simulink model "TRN_V3_2_CodeGen"  (R2022a)
settings: Solver=FixedStepAuto  StartTime=0.0  StopTime=300  FixedStep=0.04  RelTol=1e-3
PreLoadFcn:
  | load('BusStructureTRNsensor.mat');
  | addpath('C:/MAP');
InitFcn:
  | %load TRNDataBusPILS.mat
  | %addpath(genpath(cd))
  | 
  | %load('TPF_WHOLESIM_INPUT_SCENARIOS_AGCAS_N35_10E127_70.mat');
  | 
  | % Add DataBus Path
  | addpath(',,/');
  | addpath('../MAP/');
  | addpath('../MAP/MAP_DB');
  | addpath('../MAP/DVOF');
  | addpath(genpath(cd));
  | load('BusStructureTRN.mat');
undefined symbols (not defined in the file or in its folder): Altitude_INS, Latitude_INS, Longitude_INS, TRN, TRNlib
libraries: simulink_extras x23, aerolibconvert2 x6, sharedtransform x4, dspstat3 x2
(part 3 of 3)

== stateflow chart TRN_V3_2_CodeGen/TRN/ModeManagementCSU_v6 ==
  state Operation_In_Flight
    state Terrain_Referenced_Navigation [parallel]
      settings: executionOrder=1
      state TrackingCSU
        state ContinuousUpdate [parallel]
          en,du:
          [INS_Lat,INS_Lon,INS_Alt,Out_TRNDatapump.TimeTag_Prev] = TrackingCSUTimeTag(In_TRNDatapump,In_TRNInput);
          [Fmatrix,Gmatrix,M,N] = FmatGmatUpdate(INS_Lat,INS_Alt,In_TRNInput);
          [Hmat_TRN,zmat_TRN,Rmat_TRN,Hmat_GPS,zmat_GPS,Rmat_GPS, GPSflag] = ...
          TrackingCSUMeasurement(In_TRNInput,In_TRNDatapump,INS_Lat,INS_Lon,INS_Alt,M,N);
          [Out_TRNDatapump.xu, Out_Pmatrix, Out_TRNDatapump.residual, latINSErrTRN, lonINSErrTRN, altINSErrTRN,...
          Out_TRNOutput.TRNHorUncertainty, Out_TRNOutput.TRNVerticalUncertainty] ...
          = TrackingCSUEKFUpdate(In_TRNInput, zmat_TRN, zmat_GPS, Fmatrix, Hmat_TRN, Hmat_GPS, Gmatrix, In_Pmatrix, ...
          Qmatrix, Rmat_TRN, Rmat_GPS, GPSflag, Out_TRNDatapump);
          [continuousValid, Out_TRNOutput.NavigationMode]...
          = CheckValidity( Out_TRNOutput.TRNHorUncertainty, In_TRNInput.INSDataNotValid, In_TRNInput.INS_Alignment_State, ...
          In_TRNInput.GPSDataNotValid);
          [Out_TRNOutput.TRN_Ver_FlightPath_Angle] = Ver_FlightPath_Angle(In_TRNInput);
          settings: executionOrder=1
        state ContinuousValid [parallel]
          en, du:
          [Out_TRNOutput.TRNEstOfINSLatitudeErr, Out_TRNOutput.TRNEstOfINSLongitudeErr, Out_TRNOutput.TRNEstOfINSAltitudeErr, ...
          Out_TRNOutput.AircraftPositionCorrectionValid] = ValidityCheck(continuousValid, latINSErrTRN, lonINSErrTRN, altINSErrTRN);
          settings: executionOrder=2
      state AcquisitionCSU
        state Batch_On
          state StoreProfile [parallel]
            en, du: [Out_TRNDatapump.profileCnt] = StoreProfile(In_TRNInput, In_TRNDatapump);
            SetProfile(In_TRNDatapump, In_TRNInput);
            CollectProfile(Out_TRNDatapump);
            [posUpdate, Out_TRNDatapump.MAD, Out_TRNDatapump.residual] = CorrelationAnalysis(Out_TRNDatapump);
            settings: executionOrder=1
          state BatchUpdate_Valid [parallel]
            en, du:
            [Out_TRNOutput.TRNEstOfINSLatitudeErr, Out_TRNOutput.TRNEstOfINSLongitudeErr, Out_TRNOutput.TRNEstOfINSAltitudeErr, ...
            Out_TRNDatapump.profileCnt, Out_TRNOutput.NavigationMode, Out_TRNOutput.AircraftPositionCorrectionValid ] = ...
            CorrelationValid(Out_TRNDatapump, In_TRNInput, posUpdate);
            [Out_TRNOutput.TRN_Ver_FlightPath_Angle] = Ver_FlightPath_Angle(In_TRNInput);
            Out_Pmatrix = InitPmatrix();
            settings: executionOrder=2
        state Batch_Idle
          entry: Out_TRNOutput.TRNEstOfINSLatitudeErr = 0.0;
          Out_TRNOutput.TRNEstOfINSLongitudeErr = 0.0;
          Out_TRNOutput.NavigationMode = true;
          Out_TRNOutput.AircraftPositionCorrectionValid = false;
        (default) -> Batch_On
        Batch_Idle -> Batch_On : after(24, tick)
        Batch_On -> Batch_Idle : after(1, tick)
      (default) -> AcquisitionCSU
      TrackingCSU -> AcquisitionCSU : [In_TRNOutput.NavigationMode == true || ...
          | In_TRNInput.SoftResetRequest == true]
      AcquisitionCSU -> TrackingCSU : [In_TRNOutput.NavigationMode == false]
  state Flight_Idle
    en, du:
    [Out_TRNOutput.TRN_Ver_FlightPath_Angle] = Ver_FlightPath_Angle(In_TRNInput);
    Out_TRNOutput.TRN_valid = true;
    Out_TRNOutput.TRNEstOfINSLatitudeErr = 0.0;
    Out_TRNOutput.TRNEstOfINSLongitudeErr = 0.0;
    Out_TRNOutput.TRNEstOfINSAltitudeErr = 0.0;
    Out_TRNOutput.NavigationMode = false;
    Out_TRNOutput.AircraftPositionCorrectionValid = false;
  state [INS_Lat,INS_Lon,INS_Alt,TimeTag_Prev] = TrackingCSUTimeTag(In_TRNDatapump,In_TRNInput) [function]
  state [Fmatrix,Gmatrix,M,N] = FmatGmatUpdate(INS_Lat,INS_Alt,In_TRNInput) [function]
  state [Hmat_TRN,zmat_TRN,Rmat_TRN,Hmat_GPS,zmat_GPS,Rmat_GPS,GPSflag] = TrackingCSUMeasurement(In_TRNInput,In_TRNDatapump,INS_Lat,INS_Lon,INS_Alt,M,N) [function]
  state [xu,Pmatrix,residual,latINSErrTRN,lonINSErrTRN,altINSErrTRN,hUncertainty,vUncertainty] = TrackingCSUEKFUpdate(In_TRNInput,zmat_TRN,zmat_GPS,Fmatrix,Hmat_TRN,Hmat_GPS,Gmatrix,In_Pmatrix,Qmatrix,Rmat_TRN,Rmat_GPS,GPSflag,In_TRNDatapump) [function]
  state profileCnt = StoreProfile(In_TRNInput,In_TRNDatapump) [function]
  state SetProfile(In_TRNDatapump,In_TRNInput) [function]
  state CollectProfile(In_TRNDatapump) [function]
  state [posUpdate,MAD,residual] = CorrelationAnalysis(In_TRNDatapump) [function]
  state [TRNEstLatErr,TRNEstLonErr,TRNEstAltErr,profileCnt,NavigationMode,AircraftPositionCorrectionValid] = CorrelationValid(In_TRNDatapump,In_TRNInput,posUpdate) [function]
  state TRN_Ver_FlightPath_Angle = Ver_FlightPath_Angle(In_TRNInput) [function]
  state [TRNEstOfINSLatitudeErr, TRNEstOfINSLongitudeErr, TRNEstOfINSAltitudeErr, ... [function]
    AircraftPositionCorrectionValid] = ValidityCheck(continuousValid, latINSErrTRN, lonINSErrTRN, altINSErrTRN)
  (default) -> Operation_In_Flight
  Operation_In_Flight -> Flight_Idle : [In_TRNInput.WeightOnWheels == true]
  Flight_Idle -> Operation_In_Flight : [In_TRNInput.WeightOnWheels == false]
  data: In_TRNDatapump function_input Bus: TRNDatapump size=1; INS_Lat function_output; INS_Lon function_output; INS_Alt function_output; TimeTag_Prev function_output uint32 size=6; In_TRNInput function_input Bus: TRNInput size=1; INS_Lat function_input double size=1; INS_Alt function_input double size=1; Fmatrix function_output; Gmatrix function_output; In_TRNInput function_input Bus: TRNInput size=1; M function_output; N function_output; In_TRNInput function_input Bus: TRNInput size=1; In_TRNDatapump function_input Bus: TRNDatapump size=1; Hmat_TRN function_output; zmat_TRN function_output; Rmat_TRN function_output; Hmat_GPS function_output; zmat_GPS function_output size=[6 1]; Rmat_GPS function_output; INS_Lat function_input double size=1; INS_Lon function_input double size=1; INS_Alt function_input double size=1; GPSflag function_output; M function_input double size=1; N function_input double size=1; In_TRNInput function_input Bus: TRNInput size=1; zmat_TRN function_input double size=1; zmat_GPS function_input double size=[6 1]; Fmatrix function_input double size=[15 15]; Hmat_TRN function_input double size=[1 15]; Hmat_GPS function_input double size=[6 15]; Gmatrix function_input double size=[15 6]; In_Pmatrix function_input double size=[15 15]; Qmatrix function_input double size=[6 6]; Rmat_TRN function_input double size=1; Rmat_GPS function_input double size=[6 6]; GPSflag function_input uint32 size=1; In_TRNDatapump function_input Bus: TRNDatapump size=1; xu function_output; Pmatrix function_output; residual function_output; latINSErrTRN function_output; lonINSErrTRN function_output; altINSErrTRN function_output; hUncertainty function_output; vUncertainty function_output; profileCnt function_output size=1; In_TRNInput function_input Bus: TRNInput size=1 =0; In_TRNDatapump function_input Bus: TRNDatapump size=1; In_TRNDatapump function_input Bus: TRNDatapump size=1; In_TRNInput function_input Bus: TRNInput size=1; In_TRNDatapump function_input Bus: TRNDatapump size=1; In_TRNDatapump function_input Bus: TRNDatapump size=1; posUpdate function_output; MAD function_output single; residual function_output; In_TRNDatapump function_input Bus: TRNDatapump size=1; TRNEstLatErr function_output; TRNEstLonErr function_output; TRNEstAltErr function_output; In_TRNInput function_input Bus: TRNInput size=1; profileCnt function_output uint32; NavigationMode function_output boolean; AircraftPositionCorrectionValid function_output; posUpdate function_input double size=2; hUncertaintyTRN function_input; INSDataNotValid function_input; valid function_output; navigationMode function_output; INS_Alignment_State function_input; GPSDataNotValid function_input; Pmat function_output double size=[15 15]; In_TRNInput function_input Bus: TRNInput size=1; TRN_Ver_FlightPath_Angle function_output double; TRNEstOfINSLatitudeErr function_output; TRNEstOfINSLongitudeErr function_output; TRNEstOfINSAltitudeErr function_output; AircraftPositionCorrectionValid function_output boolean; continuousValid function_input boolean size=1; latINSErrTRN function_input double size=1; lonINSErrTRN function_input double size=1; altINSErrTRN function_input double size=1; In_TRNInput input Bus: TRNInput; In_TRNOutput input Bus: TRNOutput; In_TRNDatapump input Bus: TRNDatapump; In_Pmatrix input double size=[15 15]; Out_TRNOutput output Bus: TRNOutput; Out_TRNDatapump output Bus: TRNDatapump; Qmatrix input double size=[6 6]; lonINSErrTRN local double; latINSErrTRN local double; altINSErrTRN local double; continuousValid local boolean; Out_Pmatrix output double size=[15 15]; posUpdate local; Fmatrix local; Hmat_TRN local; Gmatrix local; zmat_GPS local; Rmat_TRN local; Hmat_GPS local; Rmat_GPS local; zmat_TRN local; INS_Alt local; INS_Lat local; INS_Lon local; GPSflag local; N local; M local
  function [valid, navigationMode] = CheckValidity(hUncertaintyTRN, INSDataNotValid, INS_Alignment_State, GPSDataNotValid):
    | function [valid, navigationMode] = CheckValidity(hUncertaintyTRN, INSDataNotValid, INS_Alignment_State, GPSDataNotValid)
    | 
    | persistent invalidCnt
    | if(isempty(invalidCnt))
    |     invalidCnt = 0;
    | end
    | 
    | 
    | if GPSDataNotValid == true
    |     % if(hUncertaintyTRN > (256))
    | %     if(hUncertaintyTRN > (256 / (6378000 * 25))) || (INSDataNotValid == true) || INS_Alignment_State == false
    |     if(hUncertaintyTRN > (256)) || (INSDataNotValid == true) || INS_Alignment_State == false
    |         valid = false;
    |         invalidCnt = invalidCnt + 1;
    |     else
    |         valid = true;
    |         invalidCnt = 0;
    |     end
    | else
    |     if(hUncertaintyTRN > 256) || (INSDataNotValid == true)
    |         valid = false;
    |         invalidCnt = invalidCnt + 1;
    |     else
    |         valid = true;
    |         invalidCnt = 0;
    |     end
    | end
    | 
    | if GPSDataNotValid == true
    |     if (invalidCnt > 50) || (INSDataNotValid == true)
    |         navigationMode = true;        % Acq CSU
    |     else
    |         navigationMode = false;       % Track CSU
    |     end
    | else
    |     if (invalidCnt > 50)
    |         navigationMode = true;        % Acq CSU
    |     else
    |         navigationMode = false;       % Track CSU
    |     end
    | end
    | if navigationMode == true
    |     invalidCnt = 0;
    | end
    | end
  function Pmat = InitPmatrix:
    | function Pmat = InitPmatrix()
    | 
    | R0      = 6378000;
    | 
    | attBias = [0 0 0];
    | velBias = [0 0 0];
    | posBias = [10 10 13.3] .* [1/R0 1/R0 1];
    | gyroBias = [0.4848e-6 0.4848e-6 0.4848e-6];
    | accBias = [2.9430e-4 2.9430e-4 2.9430e-4];
    | 
    | Pmat = diag([attBias velBias posBias gyroBias accBias].^2);
    | 
    | end

== matlab function TRN_V3_2_CodeGen/TRN/ModeManagementCSU_v6/CollectProfile/CollectProfile function ==
  data: hDEM output; batchProfile output; batchProfile input; profileCnt input; gridSize input; resolution input; gridRes input
function [hDEM,batchProfile]  = CollectProfile(batchProfile, profileCnt, gridSize, resolution, gridRes)

latTemp     = 0;
lonTemp     = 0;
hDEM        = 0;


for i = -gridSize : gridSize
    for j = -gridSize : gridSize
        
        latTemp = batchProfile(((profileCnt-1)*(3+(gridSize+gridSize+1)*(gridSize+gridSize+1))) + 2) + i*gridRes*resolution;
        lonTemp = batchProfile(((profileCnt-1)*(3+(gridSize+gridSize+1)*(gridSize+gridSize+1))) + 3) + j*gridRes*resolution;
        hDEM    = coder.ceval('MAPGetTerrainHeight', latTemp*180/pi, lonTemp*180/pi);

        batchProfile(((profileCnt-1)*(3+(gridSize+gridSize+1)*(gridSize+gridSize+1))) + 3 + ((i + gridSize) * (gridSize+gridSize+1)) + (j + gridSize + 1)) = abs(batchProfile(((profileCnt-1)*(3+(gridSize+gridSize+1)*(gridSize+gridSize+1))) + 1) - hDEM );   
    end
end



end

== matlab function TRN_V3_2_CodeGen/TRN/ModeManagementCSU_v6/CorrelationAnalysis/CorrelationAnalysis function ==
  data: batchProfile input; profileCnt input; posUpdate output; MAD output; gridSize input; residual output; resolution input; gridRes input
function [posUpdate, MAD, residual] = CorrelationAnalysis(batchProfile, profileCnt, gridSize, resolution, gridRes)

MAD         = single(0);
bestIdx     = [-999 -999];
posUpdate   = zeros(2,1);
MADTemp     = 9999*ones(1,8000);
sum         = 0;

for i = 1 : (gridSize+gridSize+1) * (gridSize+gridSize+1)
    sum = 0;
    for j = 1 : profileCnt
        sum = sum + batchProfile(((j-1)*(3+(gridSize+gridSize+1)*(gridSize+gridSize+1))) + (i+3));
    end
    
    MADTemp(1,i) = sum/single(profileCnt);
    
end

[minMAD, minIdx] = min(MADTemp);
MAD = single(minMAD);
bestIdx(1) = floor(minIdx/(gridSize+gridSize+1));
bestIdx(2) = minIdx - (bestIdx(1) * (gridSize+gridSize+1));

if bestIdx(2) == 0
    bestIdx(1) = bestIdx(1) - 1;
    bestIdx(2) = (gridSize+gridSize);
end
%
bestIdx(1) = bestIdx(1) - gridSize;
bestIdx(2) = bestIdx(2) - gridSize - 1;
posUpdate(1) = bestIdx(1)*gridRes*resolution;
posUpdate(2) = bestIdx(2)*gridRes*resolution;

residual = double(MAD);

end

== matlab function TRN_V3_2_CodeGen/TRN/Terrain_Func/Terrain_roughness ==
  data: Lat input; Lon input; R output
function R = Terrain_roughness(Lat, Lon)

lat2m = 110961.7060516;
lon2m = 89476.51124;

d_Lat = 90/lat2m; d_Lon = 90/lon2m;
d = 90;

A=0.0; B=0.0; C=0.0; D=0.0; E=0.0; F=0.0; G=0.0; H=0.0; I=0.0; 

A = coder.ceval('MAPGetTerrainHeight', Lat+d_Lat, Lon-d_Lon);
B = coder.ceval('MAPGetTerrainHeight', Lat+d_Lat, Lon);
C = coder.ceval('MAPGetTerrainHeight', Lat+d_Lat, Lon+d_Lon);
D = coder.ceval('MAPGetTerrainHeight', Lat, Lon-d_Lon);
E = coder.ceval('MAPGetTerrainHeight', Lat, Lon);
F = coder.ceval('MAPGetTerrainHeight', Lat, Lon+d_Lon);
G = coder.ceval('MAPGetTerrainHeight', Lat-d_Lat, Lon-d_Lon);
H = coder.ceval('MAPGetTerrainHeight', Lat-d_Lat, Lon);
I = coder.ceval('MAPGetTerrainHeight', Lat-d_Lat, Lon+d_Lon);

SLP_CR=((C+F+I)-(A+D+G))/(6*d);
SLP_DR=((A+B+C)-(G+H+I))/(6*d);

mean_R=((mean(SLP_CR)-mean(SLP_DR))/2)^2;
std_R=((std(SLP_CR)^2)+(std(SLP_DR)^2))/2;

R=sqrt(mean_R+std_R)*100;

end

== matlab function TRN_V3_2_CodeGen/TRN/ModeManagementCSU_v6/Ver_FlightPath_Angle/FlightPath_Angle ==
  data: vNED input; TRN_Ver_FlightPath_Angle output
function TRN_Ver_FlightPath_Angle  = FlightPath_Angle(vNED)

vN = vNED(1);
vE = vNED(2);
vD = vNED(3);

TRN_Ver_FlightPath_Angle = atan(-vD/sqrt(vN^2+vE^2));
